simulink model "modeloSimulinkRelayAutotuningAMIGO"  (R2019a)
settings: Solver=VariableStepAuto  StartTime=0.0  StopTime=600  RelTol=1e-3
libraries: dspsrcs4 x1
settings Model: Creator=Laura  LastModifiedBy=Laura

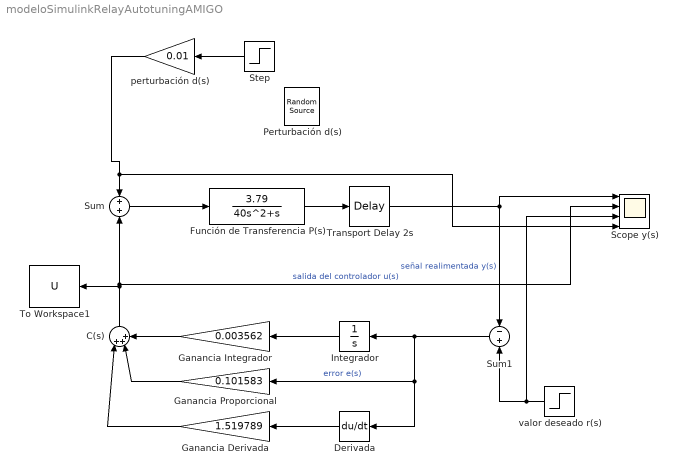
== system modeloSimulinkRelayAutotuningAMIGO ==
  " C(s)" : Sum  Inputs=|+++
  Derivada : Derivative
  Función de Transferencia P(s) : TransferFcn  Numerator=[3.79]  Denominator=[40 1 0]
  Ganancia Derivada : Gain  Gain=1.519789
  Ganancia Integrador : Gain  Gain=0.003562
  Ganancia Proporcional : Gain  Gain=0.101583
  Integrador : Integrator
  "Perturbación d(s) " : dspsrcs4/Random Source  SrcType=Uniform  NormMethod=Ziggurat  CltLength=12  MinVal=0  MaxVal=1  MeanVal=0  VarVal=1  RepMode=Not repeatable  rawSeed=1  IsInherit=off  SampMode=Discrete  SampTime=1  SampFrame=1  DataType=Double  OutComplex=Real  OutputFrames=off
  Scope y(s) : Scope  NumInputPorts=4
  Step : Step  Time=300  SampleTime=0
  Sum : Sum
  Sum1 : Sum  Inputs=-+
  To Workspace1 : ToWorkspace  VariableName=U  SampleTime=-1
      settings: Save2DSignal=2-D array (concatenate along first dimension)
  Transport Delay 2s : TransportDelay  DelayTime=2
  perturbación d(s) : Gain  Gain=0.01
  valor deseado r(s) : Step  Time=300  Before=0.32  After=0.32  SampleTime=0
  wires:
  perturbación d(s)/1 -> Sum/1, Scope y(s)/4
  valor deseado r(s)/1 -> Scope y(s)/3, Sum1/2
  Sum1/1 -> Ganancia Proporcional/1, Derivada/1, Integrador/1  "error e(s)"
  Integrador/1 -> Ganancia Integrador/1
  Derivada/1 -> Ganancia Derivada/1
  Ganancia Integrador/1 -> " C(s)"/3
  Ganancia Proporcional/1 -> " C(s)"/2
  Ganancia Derivada/1 -> " C(s)"/1
  " C(s)"/1 -> To Workspace1/1, Sum/2, Scope y(s)/2  "salida del controlador u(s)"
  Sum/1 -> Función de Transferencia P(s)/1
  Transport Delay 2s/1 -> Scope y(s)/1, Sum1/1  "señal realimentada y(s)"
  Función de Transferencia P(s)/1 -> Transport Delay 2s/1
  Step/1 -> perturbación d(s)/1
